simulink library "StatemachineSOMANET"  (R2016b)
settings: Solver=VariableStepAuto  StartTime=0.0  StopTime=10.0  RelTol=1e-3
settings Model: Creator=Nathan  LastModifiedBy=MARCH

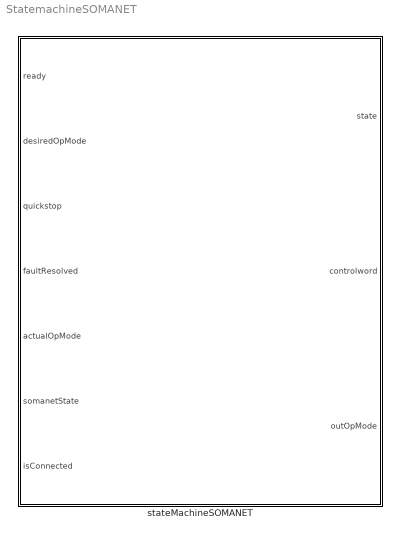
== system StatemachineSOMANET ==
  stateMachineSOMANET : Stateflow chart  TreatAsAtomicUnit=on

== stateflow chart StatemachineSOMANET/stateMachineSOMANET ==
  settings: stateMachineType=MOORE_MACHINE
  state somanet_connected
    state Initialize
      state startup_from_disconnect
        state = pending;
        controlword = SomanetControlWord.FAULT_RESET;
      state read_config
        state = startup
      state enter_tuning_mode
        outOpMode = SomanetOpmode.TUNING;
      state normal_startup
        state = pending;
        outOpMode = SomanetOpmode.NO_OPMODE;
      startup_from_disconnect -> enter_tuning_mode : [somanetState == SomanetState.SWITCH_ON_DISABLED]
      (default) -> startup_from_disconnect [order 1] : [somanetState == SomanetState.FAULT]
      normal_startup -> startup_from_disconnect [order 2] : [somanetState == SomanetState.FAULT]
      normal_startup -> enter_tuning_mode [order 1] : [somanetState == SomanetState.NOT_READY_TO_SWITCH_ON | somanetState == SomanetState.SWITCH_ON_DISABLED]
      enter_tuning_mode -> read_config : [actualOpMode == outOpMode]
      (default) -> normal_startup [order 2]
    state Operational
      state=sync
      state Switch_on_disabled
        state Choosing_control_mode
        state Sending_new_op_mode
          state Tuning_mode
            outOpMode = SomanetOpmode.TUNING;
          state None_control
            outOpMode = SomanetOpmode.NO_OPMODE;
          state Position_control
            outOpMode = SomanetOpmode.CSPOSITION;
          state Velocity_control
            outOpMode = SomanetOpmode.CSVELOCITY;
          state Torque_control
            outOpMode = SomanetOpmode.CSTORQUE;
        state Request_to_switch_on
          controlword = SomanetControlWord.SHUTDOWN; %also startup
        (default) -> Choosing_control_mode
        Choosing_control_mode -> Tuning_mode [order 4] : [desiredOpMode == SomanetOpmode.TUNING]
        Choosing_control_mode -> None_control [order 5] : [desiredOpMode == SomanetOpmode.NO_OPMODE]
        Choosing_control_mode -> Velocity_control [order 2] : [desiredOpMode == SomanetOpmode.CSVELOCITY]
        Choosing_control_mode -> Torque_control [order 3] : [desiredOpMode ==SomanetOpmode.CSTORQUE]
        Choosing_control_mode -> Position_control [order 1] : [desiredOpMode == SomanetOpmode.CSPOSITION]
        Sending_new_op_mode -> Request_to_switch_on : [outOpMode ~= SomanetOpmode.TUNING && actualOpMode == outOpMode]
      state Graceful_opmode_switch
        state graceful_switch_step_2
          controlword = SomanetControlWord.DISABLE_SWITCH_ON;
        state graceful_switch_step_1
          controlword = SomanetControlWord.SHUTDOWN;
        graceful_switch_step_1 -> graceful_switch_step_2 : [somanetState == SomanetState.READY_TO_SWITCH_ON]
      state Ready_to_switch_on
        controlword = SomanetControlWord.SWITCH_ON;
      state Quick_stop_active_desired
        controlword = SomanetControlWord.QUICK_STOP;
      state Operation_enabled
      (default) -> Switch_on_disabled
      Request_to_switch_on -> Ready_to_switch_on : [(somanetState==SomanetState.READY_TO_SWITCH_ON) && quickstop==0]
      Quick_stop_active_desired -> Switch_on_disabled : [somanetState == SomanetState.SWITCH_ON_DISABLED]
      graceful_switch_step_2 -> Switch_on_disabled : [somanetState == SomanetState.SWITCH_ON_DISABLED]
      Ready_to_switch_on -> Operation_enabled : [somanetState == SomanetState.OPERATION_ENABLED]
      Operation_enabled -> graceful_switch_step_1 [order 2] : [desiredOpMode ~= outOpMode]
      Operation_enabled -> Quick_stop_active_desired [order 1] : [quickstop == 1]
    state Fault
      state = fault
      state Fault
      state Fault_remove_desired
        controlword = SomanetControlWord.FAULT_RESET;
      state Waiting_for_resolve
        controlword = SomanetControlWord.SWITCH_ON;
      (default) -> somanet_connected.Fault.Fault
      somanet_connected.Fault.Fault -> Fault_remove_desired : [faultResolved ==1]
      Waiting_for_resolve -> Fault_remove_desired [order 2] : [faultResolved == 1]
      Fault_remove_desired -> Waiting_for_resolve [order 2] : [faultResolved == 0]
    state TuningMode
      state Tuning
        state = tuning
      state Op_desired
        outOpMode = SomanetOpmode.NO_OPMODE
      (default) -> Tuning
      Tuning -> Op_desired : [desiredOpMode ~= SomanetOpmode.TUNING]
    (default) -> Initialize
    Operational -> somanet_connected.Fault [order 1] : [somanetState == SomanetState.FAULT | somanetState == SomanetState.FAULT_REACTION_ACTIVE]
    Operational -> TuningMode [order 2] : [actualOpMode == SomanetOpmode.TUNING]
    TuningMode -> Operational : [actualOpMode ~= SomanetOpmode.TUNING]
    Waiting_for_resolve -> Operational [order 1] : [somanetState == SomanetState.SWITCH_ON_DISABLED | somanetState == SomanetState.OPERATION_ENABLED]
    Fault_remove_desired -> Operational [order 1] : [somanetState == SomanetState.SWITCH_ON_DISABLED | somanetState == SomanetState.OPERATION_ENABLED]
    read_config -> Operational : [ready == 1]
  state model_start
    state = pending
  state somanet_disconnected
    state = disconnected
  (default) -> model_start
  model_start -> somanet_connected : [isConnected==1]
  somanet_disconnected -> somanet_connected : [isConnected==1]
  somanet_connected -> somanet_disconnected : [isConnected==0]
  data: state output Enum: SomanetControlState; ready input; desiredOpMode input Enum: SomanetOpmode; quickstop input double; faultResolved input; actualOpMode input Enum: SomanetOpmode; somanetState input Enum: SomanetState; controlword output Enum: SomanetControlWord; outOpMode output Enum: SomanetOpmode; isConnected input
